simulink model "filter_crop"  (R2017a)
settings: Solver=VariableStepAuto  StartTime=0.0  StopTime=10.0  RelTol=1e-3
undefined symbols (not defined in the file): Rec, SDTV
libraries: visionconversions x2, dspvision x1
settings Model: Creator=Pection  LastModifiedBy=Pection

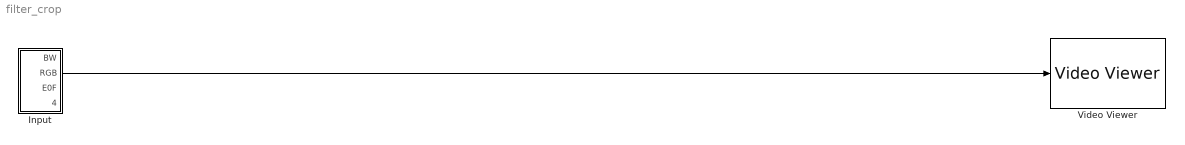
== system filter_crop ==
  "Input " : Subsystem
  Video Viewer : VideoViewer  FigPos=[1 1038 1920 938]
  wires:
  "Input "/2("RGB ") -> Video Viewer/1

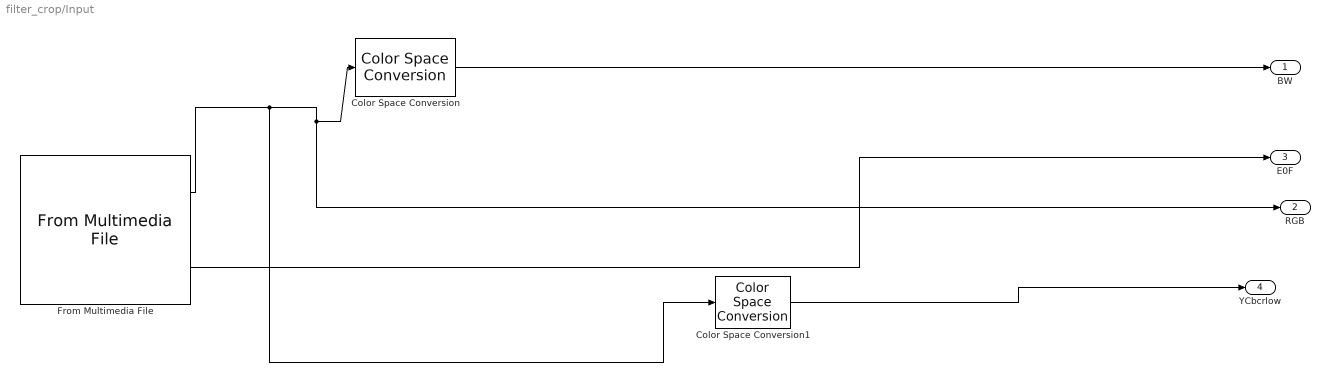
== system filter_crop/Input  ==
  Color Space Conversion : visionconversions/Color Space  Conversion  conversion=Obsolete  conversionActive=R'G'B' to intensity  wp_str=D65  rec=Rec. 601 (SDTV)  sys=1125/60/2:1  imagePorts=One multidimensional signal
      settings: SourceProductName=Computer Vision System Toolbox
  Color Space Conversion1 : visionconversions/Color Space  Conversion  conversion=Obsolete  conversionActive=R'G'B' to Y'CbCr  wp_str=D65  rec=Rec. 601 (SDTV)  sys=1125/60/2:1  imagePorts=One multidimensional signal
      settings: SourceProductName=Computer Vision System Toolbox
  From Multimedia File : dspvision/From Multimedia File  inputFilename=C:\MatlabCode\amas_2017\test_stright.webm  loop=on  numPlays=inf  outputStreams=Video only  videoDataType=single  audioDataType=int16  inheritSampleTime=off  userDefinedSampleTime=1/30  noAudioOutput=off  isIntensityVideo=off  fourcc=RGB  colorVideoFormat=One multidimensional signal  outputEOF=on  dataOrg=Column-major  audioFrameSize=1024  computeAudioFrameSize=off  outSamplingMode=Sample based
      settings: SourceProductBaseCode=VP
  BW : Outport
  "RGB " : Outport  Port=2
  E0F : Outport  Port=3
  "YCbcrlow " : Outport  Port=4
  wires:
  Color Space Conversion/1 -> BW/1
  From Multimedia File/2 -> E0F/1
  From Multimedia File/1 -> Color Space Conversion1/1, "RGB "/1, Color Space Conversion/1
  Color Space Conversion1/1 -> "YCbcrlow "/1
